simulink model "RocketFlightSimTest"  (R2020b)
settings: Solver=ode4  StartTime=0.0  StopTime=10  FixedStep=0.01  RelTol=1e-3
settings Model: Creator=bowen  LastModifiedBy=bowen

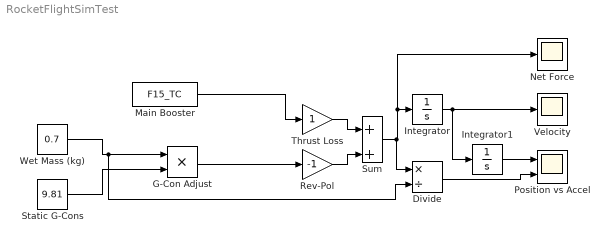
== system RocketFlightSimTest ==
  Divide : Product  Inputs=*/
  G-Con Adjust : Product
  Integrator : Integrator
  Integrator1 : Integrator
  Main Booster : FromWorkspace  VariableName=F15_TC
  Net Force : Scope
  Position vs Accel : Scope  NumInputPorts=2
  Rev-Pol : Gain  Gain=-1
  Static G-Cons : Constant  Value=9.81
  Sum : Sum  Inputs=|++
  Thrust Loss : Gain
  Velocity : Scope
  Wet Mass (kg) : Constant  Value=0.7
  wires:
  Static G-Cons/1 -> G-Con Adjust/2
  Wet Mass (kg)/1 -> Divide/2, G-Con Adjust/1
  Main Booster/1 -> Thrust Loss/1
  Thrust Loss/1 -> Sum/1
  G-Con Adjust/1 -> Rev-Pol/1
  Rev-Pol/1 -> Sum/2
  Integrator1/1 -> Position vs Accel/1
  Integrator/1 -> Velocity/1, Integrator1/1
  Sum/1 -> Divide/1, Net Force/1, Integrator/1
  Divide/1 -> Position vs Accel/2
